simulink model "e9_sf_slswitch"  (R2020a)
settings: Solver=FixedStepAuto  StartTime=0.0  StopTime=options.T_train  FixedStep=options.dt  MaxStep=.2  RelTol=1e-3
model workspace (MAT data in the model file):
  PID_TRESH = 0.3
undefined symbols (not defined in the file or in its folder): DiscIntNeverNeededParam, options
libraries: neural x72, simulink x3
(part 2 of 3)

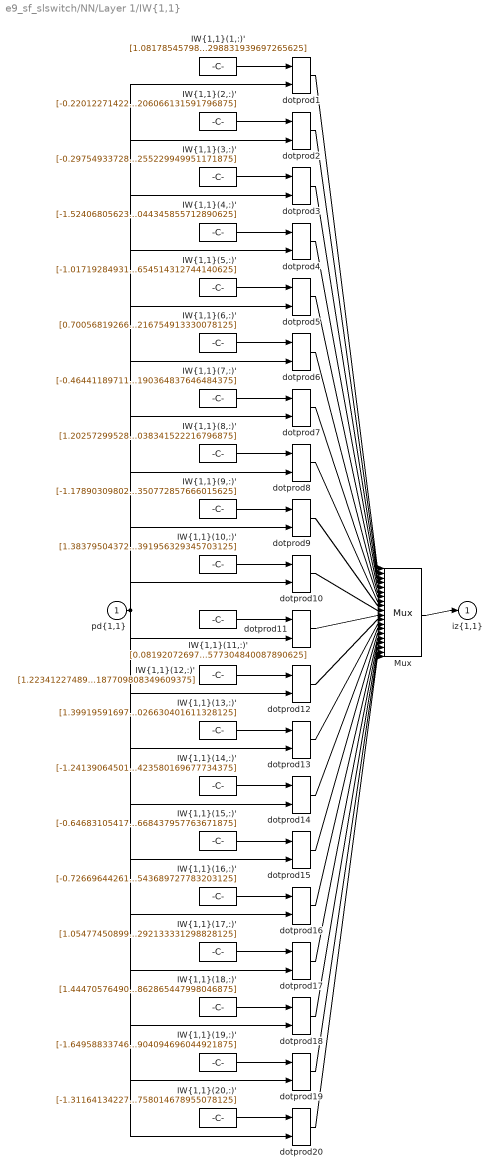
== system e9_sf_slswitch/NN/Layer 1/IW{1,1} ==
  "pd{1,1}" : Inport  PortDimensions=6
      mask Display: e = 0.06;c1 = [120 230 180]/255;c2 = ([120 230 180]+0)/(256+128);c3 = ([120 230 180]+128)/(256+128);patch([0 1 1 0],[0 0 1 1],c1);patch([0 1 1 1-e 1-e 0+e],[0 0 1 1-e 0+e 0+e],c2);patch([0 0 1 1-e 0+e 0+e],[0 1 1 1-e 1-e 0+e],c3);plot([0 1 1 0 0],[0 0 1 1 0]);
  "IW{1,1}(1,:)'" : Constant  Value=[1.0817854579839341067071245561237446963787078857421875;-0.65914064939122762876166916612419299781322479248046875;-1.4539120842314463555311476739007048308849334716796875;-0.86294267941634306140485932701267302036285400390625;0.2177432040734797735748173863612464629113674163818359375;-0.69373383704116042824949772693798877298831939697265625]
      mask Display: e = 0.06;c1 = [120 150 230]/255;c2 = ([120 150 230]+0)/383;c3 = ([120 150 230]+128)/383;patch([0 1 1 0],[0 0 1 1],c1);patch([0 1 1 1-e 1-e 0+e],[0 0 1 1-e 0+e 0+e],c2);patch([0 0 1 1-e 0+e 0+e],[0 1 1 1-e 1-e 0+e],c3);plot([0 1 1 0 0],[0 0 1 1 0]);disp('Weights');
  "IW{1,1}(10,:)'" : Constant  Value=[1.3837950437243915491336565537494607269763946533203125;0.55944885066554828068063898172113113105297088623046875;-0.0176901157466400026085917573936967528425157070159912109375;0.2068426701552374680215251601111958734691143035888671875;-0.438819528851138562774991669357405044138431549072265625;0.492641586404712672475625367951579391956329345703125]
      mask Display: e = 0.06;c1 = [120 150 230]/255;c2 = ([120 150 230]+0)/383;c3 = ([120 150 230]+128)/383;patch([0 1 1 0],[0 0 1 1],c1);patch([0 1 1 1-e 1-e 0+e],[0 0 1 1-e 0+e 0+e],c2);patch([0 0 1 1-e 0+e 0+e],[0 1 1 1-e 1-e 0+e],c3);plot([0 1 1 0 0],[0 0 1 1 0]);disp('Weights');
  "IW{1,1}(11,:)'" : Constant  Value=[0.08192072697890644128460024830928887240588665008544921875;-1.1845490216175988962277187965810298919677734375;-0.4757668709031908083062489822623319923877716064453125;-1.7649993657396925161862100139842368662357330322265625;-0.22523156626923424017405750419129617512226104736328125;-0.264773764308994297156374386759125627577304840087890625]
      mask Display: e = 0.06;c1 = [120 150 230]/255;c2 = ([120 150 230]+0)/383;c3 = ([120 150 230]+128)/383;patch([0 1 1 0],[0 0 1 1],c1);patch([0 1 1 1-e 1-e 0+e],[0 0 1 1-e 0+e 0+e],c2);patch([0 0 1 1-e 0+e 0+e],[0 1 1 1-e 1-e 0+e],c3);plot([0 1 1 0 0],[0 0 1 1 0]);disp('Weights');
  "IW{1,1}(12,:)'" : Constant  Value=[1.2234122748900606580946259782649576663970947265625;0.90710088573223146557467089223791845142841339111328125;1.4176432864784971332738905402948148548603057861328125;-1.1020871932910762946988825206062756478786468505859375;0.838005161133941189888219014392234385013580322265625;0.8495506223937530076995017225272022187709808349609375]
      mask Display: e = 0.06;c1 = [120 150 230]/255;c2 = ([120 150 230]+0)/383;c3 = ([120 150 230]+128)/383;patch([0 1 1 0],[0 0 1 1],c1);patch([0 1 1 1-e 1-e 0+e],[0 0 1 1-e 0+e 0+e],c2);patch([0 0 1 1-e 0+e 0+e],[0 1 1 1-e 1-e 0+e],c3);plot([0 1 1 0 0],[0 0 1 1 0]);disp('Weights');
  "IW{1,1}(13,:)'" : Constant  Value=[1.399195916978347664638704372919164597988128662109375;1.0543963732768075747259217678220011293888092041015625;-0.61242851620136551371587074754643253982067108154296875;-0.08090178336701096817318301646082545630633831024169921875;0.51648068034945382454026230334420688450336456298828125;1.5094087959769553197730829197098501026630401611328125]
      mask Display: e = 0.06;c1 = [120 150 230]/255;c2 = ([120 150 230]+0)/383;c3 = ([120 150 230]+128)/383;patch([0 1 1 0],[0 0 1 1],c1);patch([0 1 1 1-e 1-e 0+e],[0 0 1 1-e 0+e 0+e],c2);patch([0 0 1 1-e 0+e 0+e],[0 1 1 1-e 1-e 0+e],c3);plot([0 1 1 0 0],[0 0 1 1 0]);disp('Weights');
  "IW{1,1}(14,:)'" : Constant  Value=[-1.2413906450164489125853606310556642711162567138671875;-0.07148128728522797070699112964575760997831821441650390625;-1.1908443921462390502341577303013764321804046630859375;-0.67252402791310850194150816605542786419391632080078125;0.7554526128065621737306400973466224968433380126953125;2.344513112488522121878986581577919423580169677734375]
      mask Display: e = 0.06;c1 = [120 150 230]/255;c2 = ([120 150 230]+0)/383;c3 = ([120 150 230]+128)/383;patch([0 1 1 0],[0 0 1 1],c1);patch([0 1 1 1-e 1-e 0+e],[0 0 1 1-e 0+e 0+e],c2);patch([0 0 1 1-e 0+e 0+e],[0 1 1 1-e 1-e 0+e],c3);plot([0 1 1 0 0],[0 0 1 1 0]);disp('Weights');
  "IW{1,1}(15,:)'" : Constant  Value=[-0.6468310541765511789691345256869681179523468017578125;-0.91005376978878149696328136997180990874767303466796875;-1.5989873355917965103145661487360484898090362548828125;0.3798360512309317815748954672017134726047515869140625;-1.118433893066968831675467299646697938442230224609375;-0.486529952531798925985384585146675817668437957763671875]
      mask Display: e = 0.06;c1 = [120 150 230]/255;c2 = ([120 150 230]+0)/383;c3 = ([120 150 230]+128)/383;patch([0 1 1 0],[0 0 1 1],c1);patch([0 1 1 1-e 1-e 0+e],[0 0 1 1-e 0+e 0+e],c2);patch([0 0 1 1-e 0+e 0+e],[0 1 1 1-e 1-e 0+e],c3);plot([0 1 1 0 0],[0 0 1 1 0]);disp('Weights');
  "IW{1,1}(16,:)'" : Constant  Value=[-0.726696442612663862092858835239894688129425048828125;0.09496088383690969025874295539324521087110042572021484375;-1.4117620990817929538252428756095468997955322265625;0.9391625799027851773104202948161400854587554931640625;-1.27064270474037765978891911800019443035125732421875;-0.78705535751106214803485272568650543689727783203125]
      mask Display: e = 0.06;c1 = [120 150 230]/255;c2 = ([120 150 230]+0)/383;c3 = ([120 150 230]+128)/383;patch([0 1 1 0],[0 0 1 1],c1);patch([0 1 1 1-e 1-e 0+e],[0 0 1 1-e 0+e 0+e],c2);patch([0 0 1 1-e 0+e 0+e],[0 1 1 1-e 1-e 0+e],c3);plot([0 1 1 0 0],[0 0 1 1 0]);disp('Weights');
  "IW{1,1}(17,:)'" : Constant  Value=[1.0547745089979108090716408696607686579227447509765625;-0.823939776922041122730888673686422407627105712890625;-1.305340388402752349605862036696635186672210693359375;1.0315216998817084981254765807534568011760711669921875;-1.261284597330810441917492426000535488128662109375;-1.153671727942438440805972277303226292133331298828125]
      mask Display: e = 0.06;c1 = [120 150 230]/255;c2 = ([120 150 230]+0)/383;c3 = ([120 150 230]+128)/383;patch([0 1 1 0],[0 0 1 1],c1);patch([0 1 1 1-e 1-e 0+e],[0 0 1 1-e 0+e 0+e],c2);patch([0 0 1 1-e 0+e 0+e],[0 1 1 1-e 1-e 0+e],c3);plot([0 1 1 0 0],[0 0 1 1 0]);disp('Weights');
  "IW{1,1}(18,:)'" : Constant  Value=[1.444705764908709166860489858663640916347503662109375;-1.2257253148226519012808921615942381322383880615234375;0.225449010356215395756152020112494938075542449951171875;0.7568608656968105474760477591189555823802947998046875;0.967839677504264361829200424836017191410064697265625;0.0155630835997384135704901808594513568095862865447998046875]
      mask Display: e = 0.06;c1 = [120 150 230]/255;c2 = ([120 150 230]+0)/383;c3 = ([120 150 230]+128)/383;patch([0 1 1 0],[0 0 1 1],c1);patch([0 1 1 1-e 1-e 0+e],[0 0 1 1-e 0+e 0+e],c2);patch([0 0 1 1-e 0+e 0+e],[0 1 1 1-e 1-e 0+e],c3);plot([0 1 1 0 0],[0 0 1 1 0]);disp('Weights');
  "IW{1,1}(19,:)'" : Constant  Value=[-1.649588337469355625586331370868720114231109619140625;-0.636964875623221349343339170445688068866729736328125;0.6241250588622790917980864833225496113300323486328125;-0.481741954355602020054760714629082940518856048583984375;1.683158335445863684753931011073291301727294921875;0.50288264915131442034379460892523638904094696044921875]
      mask Display: e = 0.06;c1 = [120 150 230]/255;c2 = ([120 150 230]+0)/383;c3 = ([120 150 230]+128)/383;patch([0 1 1 0],[0 0 1 1],c1);patch([0 1 1 1-e 1-e 0+e],[0 0 1 1-e 0+e 0+e],c2);patch([0 0 1 1-e 0+e 0+e],[0 1 1 1-e 1-e 0+e],c3);plot([0 1 1 0 0],[0 0 1 1 0]);disp('Weights');
  "IW{1,1}(2,:)'" : Constant  Value=[-0.2201227142226721278372991719152196310460567474365234375;-0.87475635069785140363052278189570643007755279541015625;-0.333608358085691503180925110427779145538806915283203125;-1.9994975541551347486546319487388245761394500732421875;-0.27147211225772327480854073655791580677032470703125;1.3468308173331127175487154090660624206066131591796875]
      mask Display: e = 0.06;c1 = [120 150 230]/255;c2 = ([120 150 230]+0)/383;c3 = ([120 150 230]+128)/383;patch([0 1 1 0],[0 0 1 1],c1);patch([0 1 1 1-e 1-e 0+e],[0 0 1 1-e 0+e 0+e],c2);patch([0 0 1 1-e 0+e 0+e],[0 1 1 1-e 1-e 0+e],c3);plot([0 1 1 0 0],[0 0 1 1 0]);disp('Weights');
  "IW{1,1}(20,:)'" : Constant  Value=[-1.3116413422756438844629656159668229520320892333984375;1.10521705103656842084092204459011554718017578125;0.4534552542370693384299329409259371459484100341796875;0.6861050817757308184496878311620093882083892822265625;0.51898892269949248312599365817732177674770355224609375;0.89706092037183104981323822357808239758014678955078125]
      mask Display: e = 0.06;c1 = [120 150 230]/255;c2 = ([120 150 230]+0)/383;c3 = ([120 150 230]+128)/383;patch([0 1 1 0],[0 0 1 1],c1);patch([0 1 1 1-e 1-e 0+e],[0 0 1 1-e 0+e 0+e],c2);patch([0 0 1 1-e 0+e 0+e],[0 1 1 1-e 1-e 0+e],c3);plot([0 1 1 0 0],[0 0 1 1 0]);disp('Weights');
  "IW{1,1}(3,:)'" : Constant  Value=[-0.297549337283375958662645643926225602626800537109375;-0.293318664578050392055530437573906965553760528564453125;-1.015347132735341606490919730276800692081451416015625;1.418636391792859274829652349581010639667510986328125;-1.2804949341338061064021758284070529043674468994140625;-1.0677968400746677968271569625358097255229949951171875]
      mask Display: e = 0.06;c1 = [120 150 230]/255;c2 = ([120 150 230]+0)/383;c3 = ([120 150 230]+128)/383;patch([0 1 1 0],[0 0 1 1],c1);patch([0 1 1 1-e 1-e 0+e],[0 0 1 1-e 0+e 0+e],c2);patch([0 0 1 1-e 0+e 0+e],[0 1 1 1-e 1-e 0+e],c3);plot([0 1 1 0 0],[0 0 1 1 0]);disp('Weights');
  "IW{1,1}(4,:)'" : Constant  Value=[-1.524068056232008583350534536293707787990570068359375;-0.404817676606074261513867895700968801975250244140625;-0.09627620682136896201885889468030654825270175933837890625;1.5516368404688767324017817372805438935756683349609375;0.603513768060591093700395504129119217395782470703125;-1.5946246691925305416503988453769125044345855712890625]
      mask Display: e = 0.06;c1 = [120 150 230]/255;c2 = ([120 150 230]+0)/383;c3 = ([120 150 230]+128)/383;patch([0 1 1 0],[0 0 1 1],c1);patch([0 1 1 1-e 1-e 0+e],[0 0 1 1-e 0+e 0+e],c2);patch([0 0 1 1-e 0+e 0+e],[0 1 1 1-e 1-e 0+e],c3);plot([0 1 1 0 0],[0 0 1 1 0]);disp('Weights');
  "IW{1,1}(5,:)'" : Constant  Value=[-1.0171928493158277628793939584284089505672454833984375;-0.97005232935426610740847763736383058130741119384765625;-1.38777240101396248661558274761773645877838134765625;-0.0169908990697198621078189972877225955016911029815673828125;-0.31702860935426302457784686339437030255794525146484375;0.806813623887381314858657788136042654514312744140625]
      mask Display: e = 0.06;c1 = [120 150 230]/255;c2 = ([120 150 230]+0)/383;c3 = ([120 150 230]+128)/383;patch([0 1 1 0],[0 0 1 1],c1);patch([0 1 1 1-e 1-e 0+e],[0 0 1 1-e 0+e 0+e],c2);patch([0 0 1 1-e 0+e 0+e],[0 1 1 1-e 1-e 0+e],c3);plot([0 1 1 0 0],[0 0 1 1 0]);disp('Weights');
  "IW{1,1}(6,:)'" : Constant  Value=[0.70056819266371028742668158884043805301189422607421875;-1.02752651614440804195282908040098845958709716796875;1.444622867305658697745229801512323319911956787109375;-0.9426688080470275732380969202495180070400238037109375;0.3683898319007667954139151333947665989398956298828125;-0.5372537125480640884944705248926766216754913330078125]
      mask Display: e = 0.06;c1 = [120 150 230]/255;c2 = ([120 150 230]+0)/383;c3 = ([120 150 230]+128)/383;patch([0 1 1 0],[0 0 1 1],c1);patch([0 1 1 1-e 1-e 0+e],[0 0 1 1-e 0+e 0+e],c2);patch([0 0 1 1-e 0+e 0+e],[0 1 1 1-e 1-e 0+e],c3);plot([0 1 1 0 0],[0 0 1 1 0]);disp('Weights');
  "IW{1,1}(7,:)'" : Constant  Value=[-0.464411897117164629289476351914345286786556243896484375;0.806859662253385234720326479873619973659515380859375;-1.6941377777106645385885030918871052563190460205078125;1.4041348105440916160802089507342316210269927978515625;0.6258524520460986284575710669741965830326080322265625;0.3646986319135849807793192667304538190364837646484375]
      mask Display: e = 0.06;c1 = [120 150 230]/255;c2 = ([120 150 230]+0)/383;c3 = ([120 150 230]+128)/383;patch([0 1 1 0],[0 0 1 1],c1);patch([0 1 1 1-e 1-e 0+e],[0 0 1 1-e 0+e 0+e],c2);patch([0 0 1 1-e 0+e 0+e],[0 1 1 1-e 1-e 0+e],c3);plot([0 1 1 0 0],[0 0 1 1 0]);disp('Weights');
  "IW{1,1}(8,:)'" : Constant  Value=[1.20257299528406402799873831099830567836761474609375;0.62986546478137139803976651819539256393909454345703125;-1.4100031851464540633145361425704322755336761474609375;-1.0220129834007074531854186716373078525066375732421875;-1.2012927848416399267961196528631262481212615966796875;0.94467449666360170379419969322043471038341522216796875]
      mask Display: e = 0.06;c1 = [120 150 230]/255;c2 = ([120 150 230]+0)/383;c3 = ([120 150 230]+128)/383;patch([0 1 1 0],[0 0 1 1],c1);patch([0 1 1 1-e 1-e 0+e],[0 0 1 1-e 0+e 0+e],c2);patch([0 0 1 1-e 0+e 0+e],[0 1 1 1-e 1-e 0+e],c3);plot([0 1 1 0 0],[0 0 1 1 0]);disp('Weights');
  "IW{1,1}(9,:)'" : Constant  Value=[-1.17890309802952675255482972715981304645538330078125;-0.02144600246103679774822836634484701789915561676025390625;-0.848409437811170175081088018487207591533660888671875;-0.58439769260153939800517264302470721304416656494140625;-1.5202207261253477543760936896433122456073760986328125;-0.09872144223838663634751355857588350772857666015625]
      mask Display: e = 0.06;c1 = [120 150 230]/255;c2 = ([120 150 230]+0)/383;c3 = ([120 150 230]+128)/383;patch([0 1 1 0],[0 0 1 1],c1);patch([0 1 1 1-e 1-e 0+e],[0 0 1 1-e 0+e 0+e],c2);patch([0 0 1 1-e 0+e 0+e],[0 1 1 1-e 1-e 0+e],c3);plot([0 1 1 0 0],[0 0 1 1 0]);disp('Weights');
  Mux : Mux  Inputs=20
      mask Display: e = 0.06;c1 = [120 150 230]/255;c2 = ([120 150 230]+0)/383;c3 = ([120 150 230]+128)/383;patch([0 1 1 0],[0 0 1 1],c1);patch([0 1 1 1-e 1-e 0+e],[0 0 1 1-e 0+e 0+e],c2);patch([0 0 1 1-e 0+e 0+e],[0 1 1 1-e 1-e 0+e],c3);plot([0 1 1 0 0],[0 0 1 1 0]);disp('Mux');
  dotprod{1..20} (20 alike) : neural/Weight Functions/dotprod
  "iz{1,1}" : Outport
      mask Display: e = 0.06;c1 = [120 230 180]/255;c2 = ([120 230 180]+0)/(256+128);c3 = ([120 230 180]+128)/(256+128);patch([0 1 1 0],[0 0 1 1],c1);patch([0 1 1 1-e 1-e 0+e],[0 0 1 1-e 0+e 0+e],c2);patch([0 0 1 1-e 0+e 0+e],[0 1 1 1-e 1-e 0+e],c3);plot([0 1 1 0 0],[0 0 1 1 0]);
  wires:
  "IW{1,1}(1,:)'"/1 -> dotprod1/1
  "pd{1,1}"/1 -> dotprod1/2, dotprod2/2, dotprod3/2, dotprod4/2, dotprod5/2, dotprod6/2, dotprod7/2, dotprod8/2, dotprod9/2, dotprod10/2, dotprod11/2, dotprod12/2, dotprod13/2, dotprod14/2, dotprod15/2, dotprod16/2, dotprod17/2, dotprod18/2, dotprod19/2, dotprod20/2
  dotprod1/1 -> Mux/1
  "IW{1,1}(2,:)'"/1 -> dotprod2/1
  dotprod2/1 -> Mux/2
  "IW{1,1}(3,:)'"/1 -> dotprod3/1
  dotprod3/1 -> Mux/3
  "IW{1,1}(4,:)'"/1 -> dotprod4/1
  dotprod4/1 -> Mux/4
  "IW{1,1}(5,:)'"/1 -> dotprod5/1
  dotprod5/1 -> Mux/5
  "IW{1,1}(6,:)'"/1 -> dotprod6/1
  dotprod6/1 -> Mux/6
  "IW{1,1}(7,:)'"/1 -> dotprod7/1
  dotprod7/1 -> Mux/7
  "IW{1,1}(8,:)'"/1 -> dotprod8/1
  dotprod8/1 -> Mux/8
  "IW{1,1}(9,:)'"/1 -> dotprod9/1
  dotprod9/1 -> Mux/9
  "IW{1,1}(10,:)'"/1 -> dotprod10/1
  dotprod10/1 -> Mux/10
  "IW{1,1}(11,:)'"/1 -> dotprod11/1
  dotprod11/1 -> Mux/11
  "IW{1,1}(12,:)'"/1 -> dotprod12/1
  dotprod12/1 -> Mux/12
  "IW{1,1}(13,:)'"/1 -> dotprod13/1
  dotprod13/1 -> Mux/13
  "IW{1,1}(14,:)'"/1 -> dotprod14/1
  dotprod14/1 -> Mux/14
  "IW{1,1}(15,:)'"/1 -> dotprod15/1
  dotprod15/1 -> Mux/15
  "IW{1,1}(16,:)'"/1 -> dotprod16/1
  dotprod16/1 -> Mux/16
  "IW{1,1}(17,:)'"/1 -> dotprod17/1
  dotprod17/1 -> Mux/17
  "IW{1,1}(18,:)'"/1 -> dotprod18/1
  dotprod18/1 -> Mux/18
  "IW{1,1}(19,:)'"/1 -> dotprod19/1
  dotprod19/1 -> Mux/19
  "IW{1,1}(20,:)'"/1 -> dotprod20/1
  dotprod20/1 -> Mux/20
  Mux/1 -> "iz{1,1}"/1

== system e9_sf_slswitch/NN/Layer 2/Delays 1 ==
  "p{2}" : Inport  PortDimensions=20
      mask Display: e = 0.06;c1 = [120 230 180]/255;c2 = ([120 230 180]+0)/(256+128);c3 = ([120 230 180]+128)/(256+128);patch([0 1 1 0],[0 0 1 1],c1);patch([0 1 1 1-e 1-e 0+e],[0 0 1 1-e 0+e 0+e],c2);patch([0 0 1 1-e 0+e 0+e],[0 1 1 1-e 1-e 0+e],c3);plot([0 1 1 0 0],[0 0 1 1 0]);
  mux : Mux  Inputs=1
      mask Display: e = 0.06;c1 = [120 150 230]/255;c2 = ([120 150 230]+0)/383;c3 = ([120 150 230]+128)/383;patch([0 1 1 0],[0 0 1 1],c1);patch([0 1 1 1-e 1-e 0+e],[0 0 1 1-e 0+e 0+e],c2);patch([0 0 1 1-e 0+e 0+e],[0 1 1 1-e 1-e 0+e],c3);plot([0 1 1 0 0],[0 0 1 1 0]);disp('Mux')
  "pd{2,1}" : Outport
      mask Display: e = 0.06;c1 = [120 230 180]/255;c2 = ([120 230 180]+0)/(256+128);c3 = ([120 230 180]+128)/(256+128);patch([0 1 1 0],[0 0 1 1],c1);patch([0 1 1 1-e 1-e 0+e],[0 0 1 1-e 0+e 0+e],c2);patch([0 0 1 1-e 0+e 0+e],[0 1 1 1-e 1-e 0+e],c3);plot([0 1 1 0 0],[0 0 1 1 0]);
  wires:
  "p{2}"/1 -> mux/1
  mux/1 -> "pd{2,1}"/1

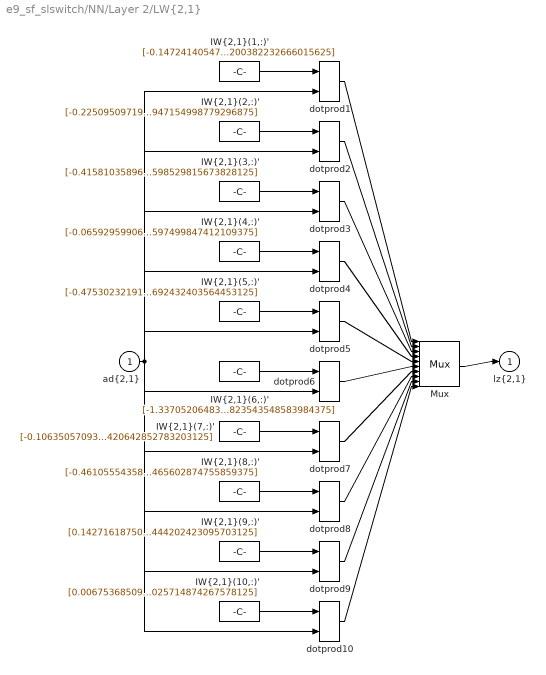
== system e9_sf_slswitch/NN/Layer 2/LW{2,1} ==
  "ad{2,1}" : Inport  PortDimensions=20
      mask Display: e = 0.06;c1 = [120 230 180]/255;c2 = ([120 230 180]+0)/(256+128);c3 = ([120 230 180]+128)/(256+128);patch([0 1 1 0],[0 0 1 1],c1);patch([0 1 1 1-e 1-e 0+e],[0 0 1 1-e 0+e 0+e],c2);patch([0 0 1 1-e 0+e 0+e],[0 1 1 1-e 1-e 0+e],c3);plot([0 1 1 0 0],[0 0 1 1 0]);
  "IW{2,1}(1,:)'" : Constant  Value=[-0.1472414054725188214955977628051186911761760711669921875;-0.2174054666444800443247942212110501714050769805908203125;0.1432666698638957736289256672534975223243236541748046875;0.31243500553130498786913449293933808803558349609375;-0.300618428587995367706753313541412353515625;-0.59337152290783123920192565492470748722553253173828125;-0.438320658255007433723449139506556093692779541015625;-0.497432537518809392285135118072503246366977691650390625;-0.317217225960222004577104826239519752562046051025390625;-0.11833226595972394512568115487738396041095256805419921875;-0.413904038860374023922616970594390295445919036865234375;-0.05439291401759217825517822575420723296701908111572265625;0.34199154888458338508172573710908181965351104736328125;0.3241148253307428728220429547945968806743621826171875;0.370814300923986817082322886562906205654144287109375;0.8413397519081515785188685185858048498630523681640625;-0.64685769485075983453725712024606764316558837890625;0.55357811263343226215738468454219400882720947265625;-0.18368456986343184578203135970397852361202239990234375;0.357233311369885397912327107405872084200382232666015625]
      mask Display: e = 0.06;c1 = [120 150 230]/255;c2 = ([120 150 230]+0)/383;c3 = ([120 150 230]+128)/383;patch([0 1 1 0],[0 0 1 1],c1);patch([0 1 1 1-e 1-e 0+e],[0 0 1 1-e 0+e 0+e],c2);patch([0 0 1 1-e 0+e 0+e],[0 1 1 1-e 1-e 0+e],c3);plot([0 1 1 0 0],[0 0 1 1 0]);disp('weights');
  "IW{2,1}(10,:)'" : Constant  Value=[0.0067536850933426380294566371276232530362904071807861328125;-0.49894962946679088933166212882497347891330718994140625;-0.467239007203976319804183958694920875132083892822265625;0.02654756634706327556028071512628230266273021697998046875;-0.58458319194564023479898651203257031738758087158203125;-0.37212757361315673687585103834862820804119110107421875;0.048499518259001707376487644296503276564180850982666015625;0.58346348773393186259994536158046685159206390380859375;-0.398918863937385015372427687907475046813488006591796875;0.150762442331681512097674158212612383067607879638671875;-0.44220289383659105997281812960864044725894927978515625;0.33750125269124542359833185400930233299732208251953125;-0.351076403120982483141432339834864251315593719482421875;0.2187294278795646196300594965578056871891021728515625;-0.53631872774196143183189633418805897235870361328125;0.28738373341429845897465611415100283920764923095703125;-0.25083434097308077159738104455755092203617095947265625;0.04202947629479052149559237250286969356238842010498046875;-0.3653835016246365086090008844621479511260986328125;-0.4093285401068715856354174320586025714874267578125]
      mask Display: e = 0.06;c1 = [120 150 230]/255;c2 = ([120 150 230]+0)/383;c3 = ([120 150 230]+128)/383;patch([0 1 1 0],[0 0 1 1],c1);patch([0 1 1 1-e 1-e 0+e],[0 0 1 1-e 0+e 0+e],c2);patch([0 0 1 1-e 0+e 0+e],[0 1 1 1-e 1-e 0+e],c3);plot([0 1 1 0 0],[0 0 1 1 0]);disp('weights');
  "IW{2,1}(2,:)'" : Constant  Value=[-0.2250950971930273103449593463665223680436611175537109375;1.4529796061393778217052386025898158550262451171875;-0.64653394985755696655616020507295615971088409423828125;-0.83337835199018694964934184099547564983367919921875;0.5630137252845608397677779066725634038448333740234375;-0.1564681148800708687662819329489138908684253692626953125;-0.38662303332659109234015204492607153952121734619140625;-0.144457803563859787931988876152900047600269317626953125;-0.202650949919479017591328329217503778636455535888671875;-0.382470720814106657226005836491822265088558197021484375;-0.62131805339441281699208730060490779578685760498046875;-0.92086272079910080901044011625344865024089813232421875;0.0080038851731276221268540638220656546764075756072998046875;0.35447779448898042442550604391726665198802947998046875;-0.62036025894475788078352707088924944400787353515625;0.27483419309341294844983849543496035039424896240234375;-0.9330227407968727515452656007255427539348602294921875;0.59159771530417082363584313497995026409626007080078125;0.75758795903734632570802887130412273108959197998046875;-0.1817390487998895576282620822894386947154998779296875]
      mask Display: e = 0.06;c1 = [120 150 230]/255;c2 = ([120 150 230]+0)/383;c3 = ([120 150 230]+128)/383;patch([0 1 1 0],[0 0 1 1],c1);patch([0 1 1 1-e 1-e 0+e],[0 0 1 1-e 0+e 0+e],c2);patch([0 0 1 1-e 0+e 0+e],[0 1 1 1-e 1-e 0+e],c3);plot([0 1 1 0 0],[0 0 1 1 0]);disp('weights');
  "IW{2,1}(3,:)'" : Constant  Value=[-0.41581035896814999563986248176661320030689239501953125;-0.737125997418619949286267001298256218433380126953125;0.229818200378771708702885234743007458746433258056640625;-0.0283744491993898097226267651649322942830622196197509765625;-0.095277561149750999991425715052173472940921783447265625;0.586153023695518360369760557659901678562164306640625;-0.60015140604928518541782977990806102752685546875;-0.70193581367152280137133857351727783679962158203125;0.09040816684742815356745637700441875495016574859619140625;0.03916327815483990060219099405003362335264682769775390625;-0.025932610402670926152968178257651743479073047637939453125;-0.606144570813990757329747793846763670444488525390625;-0.79254633552560471709824696517898701131343841552734375;-0.2187915893073386908174171594509971328079700469970703125;-0.36072925058987781454789001145400106906890869140625;0.73042680471309873180274507831200025975704193115234375;0.62967811910266446862038947074324823915958404541015625;0.60996363184678570323882240700186230242252349853515625;-0.145521436317978813956841577237355522811412811279296875;0.424444817953460173942659139356692321598529815673828125]
      mask Display: e = 0.06;c1 = [120 150 230]/255;c2 = ([120 150 230]+0)/383;c3 = ([120 150 230]+128)/383;patch([0 1 1 0],[0 0 1 1],c1);patch([0 1 1 1-e 1-e 0+e],[0 0 1 1-e 0+e 0+e],c2);patch([0 0 1 1-e 0+e 0+e],[0 1 1 1-e 1-e 0+e],c3);plot([0 1 1 0 0],[0 0 1 1 0]);disp('weights');
  "IW{2,1}(4,:)'" : Constant  Value=[-0.06592959906455829466320750498198322020471096038818359375;-0.207815956271012070022408124714274890720844268798828125;0.49804803682835530054262562771327793598175048828125;0.5627618606740749651606847692164592444896697998046875;-0.91075175118373896676615686374134384095668792724609375;-0.03868691445732264089230056924861855804920196533203125;0.08551303037956371755345941210180171765387058258056640625;1.164468657432404352647381529095582664012908935546875;-0.3573715730652526900712473434396088123321533203125;0.36447402104437376380019486532546579837799072265625;0.1961779878004633881349860757836722768843173980712890625;-0.342069691203908121668320063690771348774433135986328125;0.1253506671939809413718336372767225839197635650634765625;0.44088789320569132801352907335967756807804107666015625;-0.0957066289189872632103828209437779150903224945068359375;-0.360305667940349294564583715327898971736431121826171875;0.1915723248997241723312612293739221058785915374755859375;-0.042209600694305231260994304420819389633834362030029296875;0.0185202879361547577408142473132102168165147304534912109375;0.1726508525090853785055600155828869901597499847412109375]
      mask Display: e = 0.06;c1 = [120 150 230]/255;c2 = ([120 150 230]+0)/383;c3 = ([120 150 230]+128)/383;patch([0 1 1 0],[0 0 1 1],c1);patch([0 1 1 1-e 1-e 0+e],[0 0 1 1-e 0+e 0+e],c2);patch([0 0 1 1-e 0+e 0+e],[0 1 1 1-e 1-e 0+e],c3);plot([0 1 1 0 0],[0 0 1 1 0]);disp('weights');
  "IW{2,1}(5,:)'" : Constant  Value=[-0.4753023219176117919460011762566864490509033203125;-1.10882561282755442988445793162100017070770263671875;0.646106850860360903965329271159134805202484130859375;0.367522780052631559133402561201364733278751373291015625;-0.26050536450745831462683099744026549160480499267578125;-0.17783459990565220198988072297652252018451690673828125;-0.035236230487628937557698094451552606187760829925537109375;-0.68603475944875913494769292810815386474132537841796875;0.37680847322099297880271251415251754224300384521484375;0.11834432721891478823561527633501100353896617889404296875;-0.1880634180177349901175176682954770512878894805908203125;0.399658769857221651822243302376591600477695465087890625;-0.401875856791366670162091168094775639474391937255859375;-1.4890215742568388979094606838771142065525054931640625;0.0189470585478612764396277867717799381352961063385009765625;1.0602212891346496359545881205121986567974090576171875;0.60683237404400447445596000761725008487701416015625;0.09834765972369209630077335759779089130461215972900390625;0.62461012118992254027460830911877565085887908935546875;0.2585521652993965080469251915928907692432403564453125]
      mask Display: e = 0.06;c1 = [120 150 230]/255;c2 = ([120 150 230]+0)/383;c3 = ([120 150 230]+128)/383;patch([0 1 1 0],[0 0 1 1],c1);patch([0 1 1 1-e 1-e 0+e],[0 0 1 1-e 0+e 0+e],c2);patch([0 0 1 1-e 0+e 0+e],[0 1 1 1-e 1-e 0+e],c3);plot([0 1 1 0 0],[0 0 1 1 0]);disp('weights');
  "IW{2,1}(6,:)'" : Constant  Value=[-1.3370520648357635540293131271027959883213043212890625;-0.060057261146831707188109561457167728804051876068115234375;0.217643923701760666489235518383793532848358154296875;1.21356007364061735387394946883432567119598388671875;0.2315670300850631857514372313744388520717620849609375;-0.42836669449270015075370565682533197104930877685546875;-0.692262272507658149578446682426147162914276123046875;-0.2170729886953064735610752222783048637211322784423828125;-0.32474570226429777530796627615927718579769134521484375;0.065445042586957768993016770764370448887348175048828125;-0.05002036029582114518010627080002450384199619293212890625;0.962075041987377144181436960934661328792572021484375;-0.394416556982830124322703113648458383977413177490234375;0.376591255036607897022093993655289523303508758544921875;-0.2003929089227495519143218416502350009977817535400390625;-0.8340400862300658690884347379324026405811309814453125;0.21805150973521791879505826727836392819881439208984375;0.26071698306541890577392450722982175648212432861328125;-0.42684822579272319043042216435424052178859710693359375;-0.50428884212369862183322766213677823543548583984375]
      mask Display: e = 0.06;c1 = [120 150 230]/255;c2 = ([120 150 230]+0)/383;c3 = ([120 150 230]+128)/383;patch([0 1 1 0],[0 0 1 1],c1);patch([0 1 1 1-e 1-e 0+e],[0 0 1 1-e 0+e 0+e],c2);patch([0 0 1 1-e 0+e 0+e],[0 1 1 1-e 1-e 0+e],c3);plot([0 1 1 0 0],[0 0 1 1 0]);disp('weights');
  "IW{2,1}(7,:)'" : Constant  Value=[-0.10635057093807982753208563053703983314335346221923828125;-0.6331330730827466890531241006101481616497039794921875;0.59162381302800925997331660255440510809421539306640625;0.132444011966311891992376104099093936383724212646484375;0.002696350140554991392516370751764043234288692474365234375;0.303604538996907979964134938200004398822784423828125;-0.5051890183298597403194207799970172345638275146484375;-0.1560384324586464865891599629321717657148838043212890625;0.1748698380950980124648452829205780290067195892333984375;-0.1851266603442986158345462399665848352015018463134765625;-0.06693283860990854872152766574799898080527782440185546875;0.08253000158805905150938286851669545285403728485107421875;-0.447703828961634464622676432554726488888263702392578125;1.235813780359177105339085755986161530017852783203125;-0.63635669410014361613292521724360994994640350341796875;0.07699773153348411780516613589497865177690982818603515625;-0.04129967809423618074760042873094789683818817138671875;-0.180636742242509862332866532597108744084835052490234375;-0.3600092963214625019219283785787411034107208251953125;0.23075097523484811024019336400669999420642852783203125]
      mask Display: e = 0.06;c1 = [120 150 230]/255;c2 = ([120 150 230]+0)/383;c3 = ([120 150 230]+128)/383;patch([0 1 1 0],[0 0 1 1],c1);patch([0 1 1 1-e 1-e 0+e],[0 0 1 1-e 0+e 0+e],c2);patch([0 0 1 1-e 0+e 0+e],[0 1 1 1-e 1-e 0+e],c3);plot([0 1 1 0 0],[0 0 1 1 0]);disp('weights');
  "IW{2,1}(8,:)'" : Constant  Value=[-0.4610555435859533535136733917170204222202301025390625;0.135816376752577239184205382116488181054592132568359375;-0.0631562250634684352323944267482147552073001861572265625;-0.418554401184000501867643606601632200181484222412109375;-0.97528181590980100867938062947359867393970489501953125;-0.389632636642885887834353297876077704131603240966796875;0.318250734935395962477144848890020512044429779052734375;-0.486246452597363709724476166229578666388988494873046875;0.1483831309113791963039119536915677599608898162841796875;-0.33227206491774941010675092911696992814540863037109375;-0.08701116397057724605179629406848107464611530303955078125;-0.2304840924417397018952868847918580286204814910888671875;0.36053340362521957285224516454036347568035125732421875;0.0250056716848143199827259053336092620156705379486083984375;-0.971553413612359140216767627862282097339630126953125;-0.1763667308176421200105465914020896889269351959228515625;-0.1196440341334501777925680698899668641388416290283203125;-0.1895449774000667331197433895795256830751895904541015625;-0.5863686200399087500301220643450506031513214111328125;-0.2152732881450137580880976884145638905465602874755859375]
      mask Display: e = 0.06;c1 = [120 150 230]/255;c2 = ([120 150 230]+0)/383;c3 = ([120 150 230]+128)/383;patch([0 1 1 0],[0 0 1 1],c1);patch([0 1 1 1-e 1-e 0+e],[0 0 1 1-e 0+e 0+e],c2);patch([0 0 1 1-e 0+e 0+e],[0 1 1 1-e 1-e 0+e],c3);plot([0 1 1 0 0],[0 0 1 1 0]);disp('weights');
  "IW{2,1}(9,:)'" : Constant  Value=[0.1427161875043399807960753378210938535630702972412109375;-0.40500624990171008033001953663188032805919647216796875;0.314142033512510410186990839065401814877986907958984375;-0.5853300399394731901026034392998553812503814697265625;-0.370333972251756515792209256687783636152744293212890625;-0.336344951235155675828281118810991756618022918701171875;0.29222793400638968908111792188719846308231353759765625;0.34503902009795150984672318372759036719799041748046875;-0.142450092352637780468427308733225800096988677978515625;0.63395692895351063445019690334447659552097320556640625;-0.10489880649508621923704509981689625419676303863525390625;0.5102900660092795082078964696847833693027496337890625;-0.1739099897194994193139194749164744280278682708740234375;-0.79343415716829124306741505279205739498138427734375;-0.92886770222928272122686621514731086790561676025390625;0.016201949747158127246304815116673125885426998138427734375;0.55287321178939630161863760804408229887485504150390625;0.5700392081900369500857550519867800176143646240234375;-0.60941032802065342455222207718179561197757720947265625;0.4263003163918330784554200363345444202423095703125]
      mask Display: e = 0.06;c1 = [120 150 230]/255;c2 = ([120 150 230]+0)/383;c3 = ([120 150 230]+128)/383;patch([0 1 1 0],[0 0 1 1],c1);patch([0 1 1 1-e 1-e 0+e],[0 0 1 1-e 0+e 0+e],c2);patch([0 0 1 1-e 0+e 0+e],[0 1 1 1-e 1-e 0+e],c3);plot([0 1 1 0 0],[0 0 1 1 0]);disp('weights');
  Mux : Mux  Inputs=10
      mask Display: e = 0.06;c1 = [120 150 230]/255;c2 = ([120 150 230]+0)/383;c3 = ([120 150 230]+128)/383;patch([0 1 1 0],[0 0 1 1],c1);patch([0 1 1 1-e 1-e 0+e],[0 0 1 1-e 0+e 0+e],c2);patch([0 0 1 1-e 0+e 0+e],[0 1 1 1-e 1-e 0+e],c3);plot([0 1 1 0 0],[0 0 1 1 0]);disp('Mux');
  dotprod{1..10} (10 alike) : neural/Weight Functions/dotprod
  "lz{2,1}" : Outport
      mask Display: e = 0.06;c1 = [120 230 180]/255;c2 = ([120 230 180]+0)/(256+128);c3 = ([120 230 180]+128)/(256+128);patch([0 1 1 0],[0 0 1 1],c1);patch([0 1 1 1-e 1-e 0+e],[0 0 1 1-e 0+e 0+e],c2);patch([0 0 1 1-e 0+e 0+e],[0 1 1 1-e 1-e 0+e],c3);plot([0 1 1 0 0],[0 0 1 1 0]);
  wires:
  "IW{2,1}(1,:)'"/1 -> dotprod1/1
  "ad{2,1}"/1 -> dotprod1/2, dotprod2/2, dotprod3/2, dotprod4/2, dotprod5/2, dotprod6/2, dotprod7/2, dotprod8/2, dotprod9/2, dotprod10/2
  dotprod1/1 -> Mux/1
  "IW{2,1}(2,:)'"/1 -> dotprod2/1
  dotprod2/1 -> Mux/2
  "IW{2,1}(3,:)'"/1 -> dotprod3/1
  dotprod3/1 -> Mux/3
  "IW{2,1}(4,:)'"/1 -> dotprod4/1
  dotprod4/1 -> Mux/4
  "IW{2,1}(5,:)'"/1 -> dotprod5/1
  dotprod5/1 -> Mux/5
  "IW{2,1}(6,:)'"/1 -> dotprod6/1
  dotprod6/1 -> Mux/6
  "IW{2,1}(7,:)'"/1 -> dotprod7/1
  dotprod7/1 -> Mux/7
  "IW{2,1}(8,:)'"/1 -> dotprod8/1
  dotprod8/1 -> Mux/8
  "IW{2,1}(9,:)'"/1 -> dotprod9/1
  dotprod9/1 -> Mux/9
  "IW{2,1}(10,:)'"/1 -> dotprod10/1
  dotprod10/1 -> Mux/10
  Mux/1 -> "lz{2,1}"/1

== system e9_sf_slswitch/NN/Layer 3/Delays 1 ==
  "p{3}" : Inport  PortDimensions=10
      mask Display: e = 0.06;c1 = [120 230 180]/255;c2 = ([120 230 180]+0)/(256+128);c3 = ([120 230 180]+128)/(256+128);patch([0 1 1 0],[0 0 1 1],c1);patch([0 1 1 1-e 1-e 0+e],[0 0 1 1-e 0+e 0+e],c2);patch([0 0 1 1-e 0+e 0+e],[0 1 1 1-e 1-e 0+e],c3);plot([0 1 1 0 0],[0 0 1 1 0]);
  mux : Mux  Inputs=1
      mask Display: e = 0.06;c1 = [120 150 230]/255;c2 = ([120 150 230]+0)/383;c3 = ([120 150 230]+128)/383;patch([0 1 1 0],[0 0 1 1],c1);patch([0 1 1 1-e 1-e 0+e],[0 0 1 1-e 0+e 0+e],c2);patch([0 0 1 1-e 0+e 0+e],[0 1 1 1-e 1-e 0+e],c3);plot([0 1 1 0 0],[0 0 1 1 0]);disp('Mux')
  "pd{3,2}" : Outport
      mask Display: e = 0.06;c1 = [120 230 180]/255;c2 = ([120 230 180]+0)/(256+128);c3 = ([120 230 180]+128)/(256+128);patch([0 1 1 0],[0 0 1 1],c1);patch([0 1 1 1-e 1-e 0+e],[0 0 1 1-e 0+e 0+e],c2);patch([0 0 1 1-e 0+e 0+e],[0 1 1 1-e 1-e 0+e],c3);plot([0 1 1 0 0],[0 0 1 1 0]);
  wires:
  "p{3}"/1 -> mux/1
  mux/1 -> "pd{3,2}"/1

== system e9_sf_slswitch/NN/Layer 3/LW{3,2} ==
  "ad{3,2}" : Inport  PortDimensions=10
      mask Display: e = 0.06;c1 = [120 230 180]/255;c2 = ([120 230 180]+0)/(256+128);c3 = ([120 230 180]+128)/(256+128);patch([0 1 1 0],[0 0 1 1],c1);patch([0 1 1 1-e 1-e 0+e],[0 0 1 1-e 0+e 0+e],c2);patch([0 0 1 1-e 0+e 0+e],[0 1 1 1-e 1-e 0+e],c3);plot([0 1 1 0 0],[0 0 1 1 0]);
  "IW{3,2}(1,:)'" : Constant  Value=[0.81557987013370969453518455338780768215656280517578125;-2.04926941620302027757816176745109260082244873046875;0.94682216863196322353957157247350551187992095947265625;-0.84018970904327294757507615940994583070278167724609375;-1.2623164068393653014510391585645265877246856689453125;1.120527438989593616014417420956306159496307373046875;-0.6003909192968723829153532278724014759063720703125;0.369076046722728035032190518904826603829860687255859375;0.32198139170142103804295174995786510407924652099609375;0.048798613881968523620091815473642782308161258697509765625]
      mask Display: e = 0.06;c1 = [120 150 230]/255;c2 = ([120 150 230]+0)/383;c3 = ([120 150 230]+128)/383;patch([0 1 1 0],[0 0 1 1],c1);patch([0 1 1 1-e 1-e 0+e],[0 0 1 1-e 0+e 0+e],c2);patch([0 0 1 1-e 0+e 0+e],[0 1 1 1-e 1-e 0+e],c3);plot([0 1 1 0 0],[0 0 1 1 0]);disp('weights');
  Mux : Mux  Inputs=1
      mask Display: e = 0.06;c1 = [120 150 230]/255;c2 = ([120 150 230]+0)/383;c3 = ([120 150 230]+128)/383;patch([0 1 1 0],[0 0 1 1],c1);patch([0 1 1 1-e 1-e 0+e],[0 0 1 1-e 0+e 0+e],c2);patch([0 0 1 1-e 0+e 0+e],[0 1 1 1-e 1-e 0+e],c3);plot([0 1 1 0 0],[0 0 1 1 0]);disp('Mux');
  dotprod1 : neural/Weight Functions/dotprod
  "lz{3,2}" : Outport
      mask Display: e = 0.06;c1 = [120 230 180]/255;c2 = ([120 230 180]+0)/(256+128);c3 = ([120 230 180]+128)/(256+128);patch([0 1 1 0],[0 0 1 1],c1);patch([0 1 1 1-e 1-e 0+e],[0 0 1 1-e 0+e 0+e],c2);patch([0 0 1 1-e 0+e 0+e],[0 1 1 1-e 1-e 0+e],c3);plot([0 1 1 0 0],[0 0 1 1 0]);
  wires:
  "IW{3,2}(1,:)'"/1 -> dotprod1/1
  "ad{3,2}"/1 -> dotprod1/2
  dotprod1/1 -> Mux/1
  Mux/1 -> "lz{3,2}"/1

== system e9_sf_slswitch/NN_cex_1/Layer 1/Delays 1 ==
  "p{1}" : Inport  PortDimensions=6
      mask Display: e = 0.06;c1 = [120 230 180]/255;c2 = ([120 230 180]+0)/(256+128);c3 = ([120 230 180]+128)/(256+128);patch([0 1 1 0],[0 0 1 1],c1);patch([0 1 1 1-e 1-e 0+e],[0 0 1 1-e 0+e 0+e],c2);patch([0 0 1 1-e 0+e 0+e],[0 1 1 1-e 1-e 0+e],c3);plot([0 1 1 0 0],[0 0 1 1 0]);
  mux : Mux  Inputs=1
      mask Display: e = 0.06;c1 = [120 150 230]/255;c2 = ([120 150 230]+0)/383;c3 = ([120 150 230]+128)/383;patch([0 1 1 0],[0 0 1 1],c1);patch([0 1 1 1-e 1-e 0+e],[0 0 1 1-e 0+e 0+e],c2);patch([0 0 1 1-e 0+e 0+e],[0 1 1 1-e 1-e 0+e],c3);plot([0 1 1 0 0],[0 0 1 1 0]);disp('Mux')
  "pd{1,1}" : Outport
      mask Display: e = 0.06;c1 = [120 230 180]/255;c2 = ([120 230 180]+0)/(256+128);c3 = ([120 230 180]+128)/(256+128);patch([0 1 1 0],[0 0 1 1],c1);patch([0 1 1 1-e 1-e 0+e],[0 0 1 1-e 0+e 0+e],c2);patch([0 0 1 1-e 0+e 0+e],[0 1 1 1-e 1-e 0+e],c3);plot([0 1 1 0 0],[0 0 1 1 0]);
  wires:
  "p{1}"/1 -> mux/1
  mux/1 -> "pd{1,1}"/1
